simulink model "PID_CONTROL_GRAVEDAD"  (R2024b)
settings: Solver=VariableStepAuto  StartTime=0.0  StopTime=5  RelTol=1e-3
undefined symbols (not defined in the file): X, Y, Z
libraries: sm_lib x7, nesl_utility x6
settings Model: Creator=roque  LastModifiedBy=hecto
settings SolverCC: ZeroCrossAlgorithm=Adaptive  AlgebraicLoopSolver=TrustRegion
settings DebuggingCC: IgnoredZcDiagnostic=none  UnconnectedInputMsg=warning  UnconnectedOutputMsg=warning  UnconnectedLineMsg=warning  ArithmeticOperatorsInVariantConditions=warning
settings ModelReferenceCC: EnableRefExpFcnMdlSchedulingChecks=on
settings SFSimCC: CustomCodeUndefinedFunction=UseInterfaceOnly
settings RTWCC: GPUComputeCapability=3.5  DLArmComputeVersion=19.05

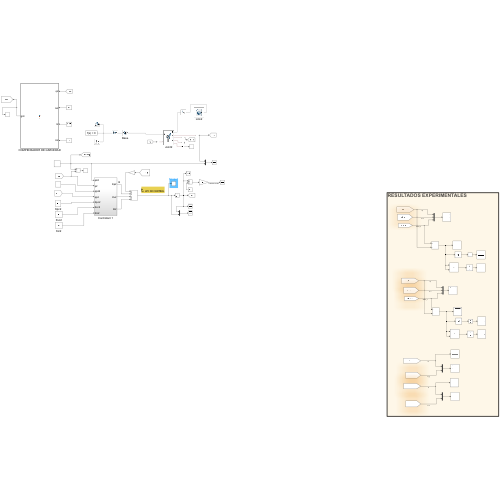
[thumbnail: Simulink's stored preview of the top-level diagram]
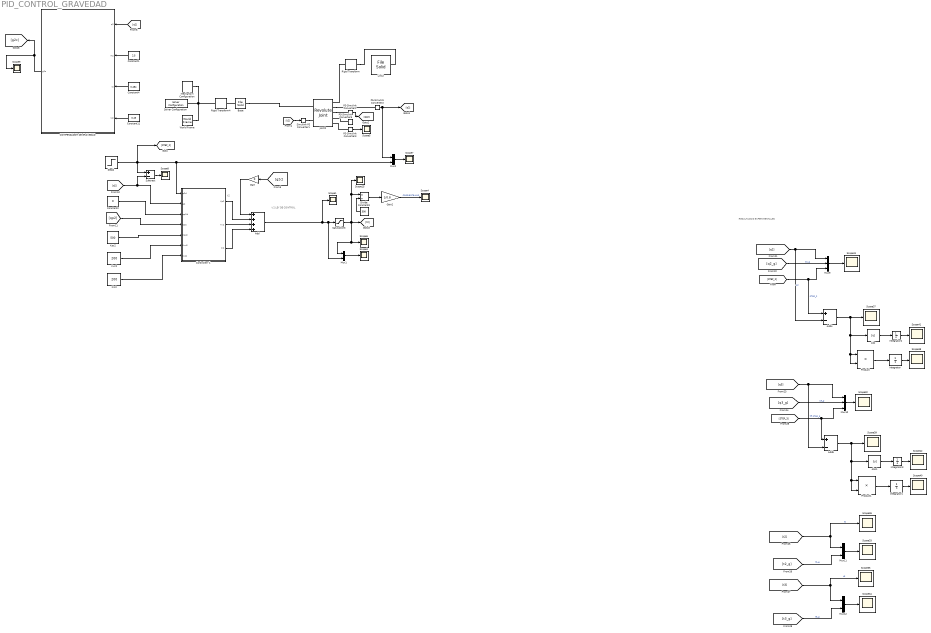
== system PID_CONTROL_GRAVEDAD ==
  note: RESULTADOS EXPERIMENTALES
  note: t 2 LEY DE CONTROL
  note: t2
  Abs : Abs  SaturateOnIntegerOverflow=off
  Abs1 : Abs  SaturateOnIntegerOverflow=off
  Add : Sum  Inputs=++++
  Add4 : Sum  Inputs=+-
  Add5 : Sum  Inputs=+-
  Base : sm_lib/Body Elements/File Solid  ExtGeomFileName=C:\Users\hecto\Desktop\OneDrive - Universidad Politécnica de Madrid\Diseño y Control Robots\Prueba Evaluacion Continua\3\SILLA\STEP\InferiorTotal.STEP  UnitType=FromFile  ExtGeomFileUnits=m  StepReaderType=HEX  ExportConvexHullGeometry=off  InertiaType=CalculateFromGeometry  BasedOnType=Density  Density=2700  DensityUnits=kg/m^3  Mass=1  MassUnits=kg  CenterOfMass=[0 0 0]  CenterOfMassUnits=m  MomentsOfInertia=[1 1 1]  MomentsOfInertiaUnits=kg*m^2  ProductsOfInertia=[0 0 0]  ProductsOfInertiaUnits=kg*m^2  GraphicType=FromGeometry  MarkerShape=Sphere  MarkerSize=10  GraphicVisPropType=SimpleVisualProperties  GraphicDiffuseColor=[1.0 0.6 0.0]  GraphicOpacity=1.0  GraphicSpecularColor=[0.5 0.5 0.5 1.0]  GraphicAmbientColor=[0.15 0.15 0.15 1.0]  GraphicEmissiveColor=[0.0 0.0 0.0 1.0]  GraphicShininess=75  DoExposeReferenceFrame=on  SerializedFrames=<Frames><Frame><Id>Frame2</Id><Value><Name>F2</Name><Origin><Source>GeometricFeature</Source><FeatureName>circular curve 27</FeatureName></Origin><PrimaryAxis><DefinedDirection>+Z</DefinedDirection><Source>GeometricFeature</Source><SourceDirection>+Z</SourceDirection><FeatureName>circular curve 27</FeatureName></PrimaryAxis><SecondaryAxis><DefinedDirection>+X</DefinedDirection><Source>ReferenceFrame</Source><SourceDirection>+X</SourceDirection><FeatureName></FeatureName></SecondaryAxis></Value></Frame></Frames>
  COMPENSADOR DE GRAVEDAD : MATLAB Function  TreatAsAtomicUnit=on
  Constant1 : Constant  Value=2.5
  Constant11 : Constant  Value=0.45
  Constant2 : Constant  Value=0
  Constant3 : Constant  Value=300
  Constant4 : Constant  Value=0.484
  Controllerr 1 : Subsystem
  Divide : Product  Inputs=*/
  Gain : Gain  Gain=0
  Gain2 : Gain  Gain=1/0.8
  Integrator{,1..3} (4 alike) : Integrator
  Joint2 : sm_lib/Joints/Revolute Joint  JointMode=Normal  CompositeWrenchDir=FollowerOnBase  CompositeWrenchFrame=BaseFrame  SenseConstraintForce=off  SenseConstraintTorque=off  SenseTotalForce=off  SenseTotalTorque=off  PositionTargetSpecify=off  PositionTargetPriority=High  PositionTargetValue=0  PositionTargetValueUnits=deg  VelocityTargetSpecify=off  VelocityTargetPriority=High  VelocityTargetValue=0  VelocityTargetValueUnits=rad/s  EquilibriumPosition=0  EquilibriumPositionUnits=deg  SpringStiffness=0  SpringStiffnessUnits=N*m/deg  DampingCoefficient=0  DampingCoefficientUnits=N*m/(deg/s)  LowerLimitSpecify=off  LowerLimitBound=-90  LowerLimitBoundUnits=deg  LowerLimitStiffness=1e4  LowerLimitStiffnessUnits=N*m/deg  LowerLimitDamping=10  LowerLimitDampingUnits=N*m/(deg/s)  LowerLimitTransitionRegionWidth=0.1  LowerLimitTransitionRegionWidthUnits=deg  UpperLimitSpecify=off  UpperLimitBound=90  UpperLimitBoundUnits=deg  UpperLimitStiffness=1e4  UpperLimitStiffnessUnits=N*m/deg  UpperLimitDamping=10  UpperLimitDampingUnits=N*m/(deg/s)  UpperLimitTransitionRegionWidth=0.1  UpperLimitTransitionRegionWidthUnits=deg  TorqueActuationMode=InputTorque  MotionActuationMode=ComputedMotion  SensePosition=on  SenseVelocity=on  SenseAcceleration=on  SenseTorqueForce=on  SenseLowerLimitTorqueForce=off  SenseUpperLimitTorqueForce=off
  Kic2 : Constant  Value=200
  Kpc2 : Constant  Value=500
  Kvc2 : Constant  Value=200
  Link2 : sm_lib/Body Elements/File Solid  ExtGeomFileName=C:\Users\hecto\Desktop\OneDrive - Universidad Politécnica de Madrid\Diseño y Control Robots\Prueba Evaluacion Continua\3\SILLA\STEP\Superior.STEP  UnitType=FromFile  ExtGeomFileUnits=m  StepReaderType=HEX  ExportConvexHullGeometry=off  InertiaType=CalculateFromGeometry  BasedOnType=Density  Density=2700  DensityUnits=kg/m^3  Mass=1  MassUnits=kg  CenterOfMass=[0 0 0]  CenterOfMassUnits=m  MomentsOfInertia=[1 1 1]  MomentsOfInertiaUnits=kg*m^2  ProductsOfInertia=[0 0 0]  ProductsOfInertiaUnits=kg*m^2  GraphicType=FromGeometry  MarkerShape=Sphere  MarkerSize=10  GraphicVisPropType=SimpleVisualProperties  GraphicDiffuseColor=[1.0 0.6 0.0]  GraphicOpacity=1  GraphicSpecularColor=[0.5 0.5 0.5 1.0]  GraphicAmbientColor=[0.15 0.15 0.15 1.0]  GraphicEmissiveColor=[0.0 0.0 0.0 1.0]  GraphicShininess=75  DoExposeReferenceFrame=off  SerializedFrames=<Frames><Frame><Id>Frame2</Id><Value><Name>F2</Name><Origin><Source>GeometricFeature</Source><FeatureName>planar surface 1</FeatureName></Origin><PrimaryAxis><DefinedDirection>+Z</DefinedDirection><Source>GeometricFeature</Source><SourceDirection>+Z</SourceDirection><FeatureName>planar surface 1</FeatureName></PrimaryAxis><SecondaryAxis><DefinedDirection>+X</DefinedDirection><Source>ReferenceFrame</Source><SourceDirection>-X</SourceDirection><FeatureName>segment 63</FeatureName></SecondaryAxis></Value></Frame></Frames>
  Mechanism Configuration : sm_lib/Utilities/Mechanism Configuration  UniformGravity=Constant  GravityVector=[0 0 -9.80665]  GravityVectorUnits=m/s^2  LinearizationDelta=0.001  JointModeTransitionNonlinearIterations=2
  Mux{1..2,11..12} (4 alike) : Mux  Inputs=2
  Mux10 : Mux  Inputs=3
  Mux9 : Mux  Inputs=3
  PS-Simulink Converter1 : nesl_utility/PS-Simulink Converter  PhysicalDomain=network_engine_domain  SubClassName=ps_output  LeftPortType=input  RightPortType=output  PseudoPeriodic=off  Frequencies=[]  VectorFormat=1-D array  Unit=1  AffineConversion=on
  PS-Simulink Converter2 : nesl_utility/PS-Simulink Converter  PhysicalDomain=network_engine_domain  SubClassName=ps_output  LeftPortType=input  RightPortType=output  PseudoPeriodic=off  Frequencies=[]  VectorFormat=1-D array  Unit=rad  AffineConversion=on
  PS-Simulink Converter3 : nesl_utility/PS-Simulink Converter  PhysicalDomain=network_engine_domain  SubClassName=ps_output  LeftPortType=input  RightPortType=output  PseudoPeriodic=off  Frequencies=[]  VectorFormat=1-D array  Unit=N*m  AffineConversion=on
  PS-Simulink Converter5 : nesl_utility/PS-Simulink Converter  PhysicalDomain=network_engine_domain  SubClassName=ps_output  LeftPortType=input  RightPortType=output  PseudoPeriodic=off  Frequencies=[]  VectorFormat=1-D array  Unit=1  AffineConversion=on
  Product : Product
  Product1 : Product
  Rigid Transform : sm_lib/Frames and Transforms/Rigid Transform  RotationMethod=StandardAxis  FollAlignAxisA=+X  BaseAlignAxisA=+Y  FollAlignAxisB=+Y  BaseAlignAxisB=+Z  RotationStandardAxis=-Z  RotationAngle=0  RotationAngleUnits=deg  RotationArbitraryAxis=[0 0 1]  RotationSequenceAxes=FollowerAxes  RotationSequence=XYX  RotationSequenceAngles=[0 0 0]  RotationSequenceAnglesUnits=deg  RotationMatrix=[1 0 0; 0 1 0; 0 0 1]  Quaternion=[1 0 0 0]  TranslationMethod=None  TranslationCartesianOffset=[0 0 0]  TranslationCartesianOffsetUnits=m  TranslationStandardAxis=+Z  TranslationStandardOffset=0  TranslationStandardOffsetUnits=m  TranslationROffset=0  TranslationROffsetUnits=m  TranslationThetaOffset=0  TranslationThetaOffsetUnits=deg  TranslationZOffset=0  TranslationZOffsetUnits=m
  Rigid Transform4 : sm_lib/Frames and Transforms/Rigid Transform  RotationMethod=AlignedAxes  FollAlignAxisA=+Y  BaseAlignAxisA=-Z  FollAlignAxisB=+X  BaseAlignAxisB=+X  RotationStandardAxis=+Z  RotationAngle=0.0  RotationAngleUnits=deg  RotationArbitraryAxis=[0 0 1]  RotationSequenceAxes=FollowerAxes  RotationSequence=XYX  RotationSequenceAngles=[0 0 0]  RotationSequenceAnglesUnits=deg  RotationMatrix=[1 0 0; 0 1 0; 0 0 1]  Quaternion=[1 0 0 0]  TranslationMethod=Cartesian  TranslationCartesianOffset=[0 0 0]  TranslationCartesianOffsetUnits=m  TranslationStandardAxis=+Z  TranslationStandardOffset=0  TranslationStandardOffsetUnits=m  TranslationROffset=0  TranslationROffsetUnits=m  TranslationThetaOffset=0  TranslationThetaOffsetUnits=deg  TranslationZOffset=0  TranslationZOffsetUnits=m
  Saturation3 : Saturate  UpperLimit=1290  LowerLimit=-1290
  Scope{1,3..9,15,31..42} (21 alike) : Scope
  Simulink-PS Converter1 : nesl_utility/Simulink-PS Converter  PhysicalDomain=network_engine_domain  SubClassName=ps_input  LeftPortType=input  RightPortType=output  PseudoPeriodic=off  Frequencies=[]  NoiseDistribution=none  NoiseParameters=[]  Unit=N*m  AffineConversion=off  FilteringAndDerivatives=filter  SimscapeFilterOrder=2  InputFilterTimeConstant=0.001  UdotUserProvided=0
  Solver Configuration : nesl_utility/Solver Configuration  PhysicalDomain=network_engine_domain  SubClassName=solver  LeftPortType=input  RightPortType=generic  Tones=[]  Harmonics=[]  SimulateNoise=off  Profile=off  UseLocalSampling=off  EnableSwitchedLinearOptims=on  FrequencyDomain=off  UseCCode=off  RelTol=0.001  AbsTol=1e-06  MinStep=1e-09  ToWorkspace=off  RevertToSquareIcSolve=off  NumHomotopyIterations=100  PhasorMode=off  PhasorModeNumHarmonics=1  ConsistencySolver=NEWTON_FTOL  IndexReductionMethod=DerivativeReplacement  DoDC=off  ResidualTolerance=1e-09  ConsistencyTolSource=GLOBAL  ConsistencyAbsTol=0.001  ConsistencyRelTol=0.001  ConsistencyTolFactor=0.001  UseLocalSolver=off  LocalSolverChoice=NE_BACKWARD_EULER_ADVANCER  ResolveIndetEquations=on  FunctionEvalNumThread=1  LocalSolverSampleTime=0.001  DoFixedCost=off  MaxNonlinIter=3  MaxModeIter=2  ComputeImpulses=off  ImpulseIterations=2  LinearAlgebra=auto  LinearAlgebraNumThread=0  EquationFormulation=NE_TIME_EF  DelaysMemoryBudget=1024  AutomaticFiltering=on  FilteringTimeConstant=0.001  PartitionStorageMethod=AS_NEEDED  PartitionMemoryBudget=1024  PartitionMethod=ROBUST  MultibodyUseLocalSolver=off  MultibodyLocalSolverChoice=ODE1  MultibodyLocalSolverSampleTime=0.001
  Step2 : Step  Time=0  After=pi/4  SampleTime=0
  Subtract : Sum  Inputs=+-
  World Frame : sm_lib/Frames and Transforms/World Frame
  wires:
  Kic2/1 -> Controllerr 1/7(Kic2)
  Controllerr 1/2(Kv2) -> Add/3
  Kvc2/1 -> Controllerr 1/6(Kvc2)
  Controllerr 1/1(Kp2) -> Add/2
  Kpc2/1 -> Controllerr 1/5(Kpc2)
  Constant2/1 -> Controllerr 1/3(qp2d)
  Constant3/1 -> Divide/2
  Controllerr 1/3(Ki2) -> Add/4
  Mux1/1 -> Scope3/1
  Divide/1 -> Gain2/1
  Gain2/1 -> Scope4/1  "CORRIENTE-AMP"
  [g2c] -> Gain/1
  Gain/1 -> Add/1
  [qp2] -> Controllerr 1/4(qp2)
  Subtract/1 -> Scope8/1
  Step2/1 -> [STEP_2], Subtract/1, Controllerr 1/1(q2d), Mux2/2
  [q2] -> Controllerr 1/2(q2), Subtract/2
  PS-Simulink Converter2/1 -> Mux2/1, [q2]
  PS-Simulink Converter1/1 -> [qp2]
  PS-Simulink Converter3/1 -> Scope5/1
  [t2] -> Simulink-PS Converter1/1
  Mux2/1 -> Scope7/1
  Constant1/1 -> COMPENSADOR DE GRAVEDAD/2(m2)
  Constant4/1 -> COMPENSADOR DE GRAVEDAD/3(I2)
  Constant11/1 -> COMPENSADOR DE GRAVEDAD/4(lc2)
  COMPENSADOR DE GRAVEDAD/1(g2c) -> [g2c], Scope9/1
  Add/1 -> Saturation3/1, Mux1/2, Scope1/1
  Saturation3/1 -> Scope6/1, Mux1/1, [t2], Scope15/1, Divide/1
  Mux9/1 -> Scope31/1
  [q2_g] -> Mux9/2  "q2_g"
  [q2] -> Add4/2, Mux9/1  "q2"
  [q3] -> Add5/2, Mux10/1  "q3"
  [q3_g] -> Mux10/2  "q3_g"
  Mux10/1 -> Scope32/1
  Mux11/1 -> Scope33/1
  [t2_g] -> Mux11/2  "t2_g"
  [t2] -> Mux11/1, Scope36/1  "t2"
  [t3] -> Mux12/1, Scope35/1  "t3"
  [t3_g] -> Mux12/2  "t3_g"
  Mux12/1 -> Scope34/1
  [STEP_2] -> Add4/1, Mux9/3  "STEP_2"
  [STEP_3] -> Add5/1, Mux10/3  "STEP_3"
  Add4/1 -> Abs/1, Product/2, Product/1, Scope37/1
  Integrator/1 -> Scope38/1
  Integrator2/1 -> Scope41/1
  Abs/1 -> Integrator2/1
  Product/1 -> Integrator/1
  Product1/1 -> Integrator1/1
  Abs1/1 -> Integrator3/1
  Integrator3/1 -> Scope42/1
  Integrator1/1 -> Scope40/1
  Add5/1 -> Scope39/1, Product1/1, Product1/2, Abs1/1
  [q2] -> COMPENSADOR DE GRAVEDAD/1(q2)
  connections:
  Base/RConn1 -- Rigid Transform4/LConn1
  World Frame/RConn1 -- Rigid Transform4/RConn1 -- Solver Configuration/RConn1 -- Mechanism Configuration/RConn1
  Joint2/RConn3 -- PS-Simulink Converter1/LConn1
  Joint2/RConn2 -- PS-Simulink Converter2/LConn1
  PS-Simulink Converter5/LConn1 -- Joint2/RConn4
  PS-Simulink Converter3/LConn1 -- Joint2/RConn5
  Simulink-PS Converter1/RConn1 -- Joint2/LConn2
  Base/LConn1 -- Joint2/LConn1
  Rigid Transform/RConn1 -- Joint2/RConn1
  Rigid Transform/LConn1 -- Link2/LConn1

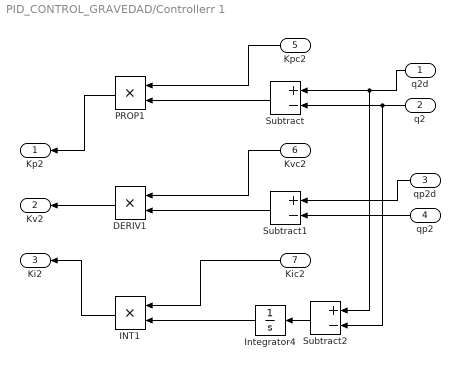
== system PID_CONTROL_GRAVEDAD/Controllerr 1 ==
  q2d : Inport
  q2 : Inport  Port=2
  qp2d : Inport  Port=3
  qp2 : Inport  Port=4
  Kpc2 : Inport  Port=5
  Kvc2 : Inport  Port=6
  Kic2 : Inport  Port=7
  DERIV1 : Product
  INT1 : Product
  Integrator4 : Integrator
  PROP1 : Product
  Subtract : Sum  Inputs=+-
  Subtract1 : Sum  Inputs=+-
  Subtract2 : Sum  Inputs=+-
  Kp2 : Outport  VectorParamsAs1DForOutWhenUnconnected=off
  Kv2 : Outport  Port=2  VectorParamsAs1DForOutWhenUnconnected=off
  Ki2 : Outport  Port=3  VectorParamsAs1DForOutWhenUnconnected=off
  wires:
  q2/1 -> Subtract2/2, Subtract/2
  qp2/1 -> Subtract1/2
  INT1/1 -> Ki2/1
  Kvc2/1 -> DERIV1/1
  qp2d/1 -> Subtract1/1
  Subtract1/1 -> DERIV1/2
  q2d/1 -> Subtract2/1, Subtract/1
  Kic2/1 -> INT1/1
  DERIV1/1 -> Kv2/1
  Subtract/1 -> PROP1/2
  PROP1/1 -> Kp2/1
  Subtract2/1 -> Integrator4/1
  Integrator4/1 -> INT1/2
  Kpc2/1 -> PROP1/1

== matlab function PID_CONTROL_GRAVEDAD/COMPENSADOR DE GRAVEDAD ==
  data: q2 input; g2c output; m2 input; I2 input; lc2 input
function g2c  = g(q2, m2, I2, lc2)

% Parametros del robot
%m2=23.902; m3=3.88;
%L2=0.45; L3=0.45; lc2=0.091;lc3=0.0229;
%I2=1.266; I3=0.093;

g2c=(m2*lc2)*9.8*sin(q2);
%G=[g2c g3c]';

%gc = [g2c;g3c];
